simulink model "bh_lag_LQI_eom_quad_include_spin_props"  (R2021b)
settings: Solver=ode23t  StartTime=0.0  StopTime=200  FixedStep=0.001  RelTol=1e-5  EnableMultiTasking=on
values from neighbouring files (symbols this model uses):
  K = [1.17115605021e-19 -1.34457008772e-16 -7.12795123873e-18 0.0431836511993 -1.6541551896e-12 -1.73191982917e-16 0.126584124772 -3.94383892487e-18 1.65419671556e-12 0.126584124772 -1.82762947107e-16 -8.51651764895e-17 ... (60 elements, 4x15)]    [OLD_bh_CONT_DES_RESULTS_LQI_quadcopter.mat]    (also in bh_CONT_DES_RESULTS_LQI_quadcopter.mat = [2.6635655919e-18 -4.41749299763e-16 -1.11640474601e-16 0.04)
undefined symbols (not defined in the file or in its folder): P_elec, P_mot, P_one_prop, P_veh, sigbuilder_block
libraries: bh_6dof_LIBRARY x21, simulink_extras x12, slpidlib x4, simulink x1
(part 1 of 2)
settings Model: Creator=bhorton  LastModifiedBy=bhorton
settings SolverCC: AlgebraicLoopSolver=TrustRegion
settings DataIOCC: SaveOutput=off  SignalLogging=off  DSMLogging=off  VisualizeSimOutput=off  SaveTime=off  ReturnWorkspaceOutputs=off
settings OptimizationCC: LifeSpan=inf
settings DebuggingCC: AllowSymbolicDim=off  SFUnexpectedBacktrackingDiag=warning  SFNoUnconditionalDefaultTransitionDiag=warning  SFExecutionAtInitializationDiag=none  SFMachineParentedDataDiag=warning  ArithmeticOperatorsInVariantConditions=warning
settings ModelReferenceCC: PropagateSignalLabelsOutOfModel=off
settings SFSimCC: SimUseLocalCustomCode=off  CustomCodeUndefinedFunction=UseInterfaceOnly
settings RTWCC: RTWUseLocalCustomCode=off
settings CodeAppCC: StateflowObjectComments=on
settings GRTTargetCC: TargetLangStandard=C89/C90 (ANSI)
settings ConfigComp: CovMetricSettings=dw  CovSaveCumulativeToWorkspaceVar=on  CovSaveSingleToWorkspaceVar=on  CovExternalEMLEnable=off

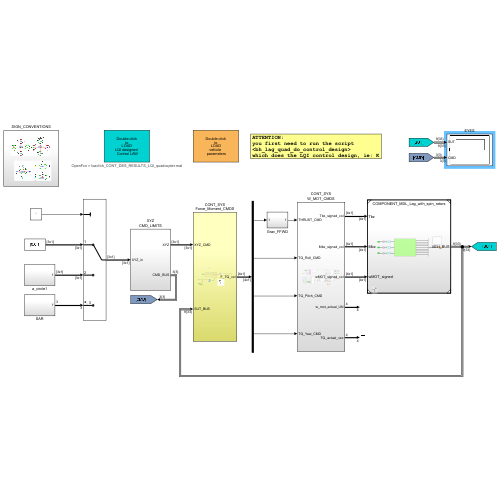
[thumbnail: Simulink's stored preview of the top-level diagram]
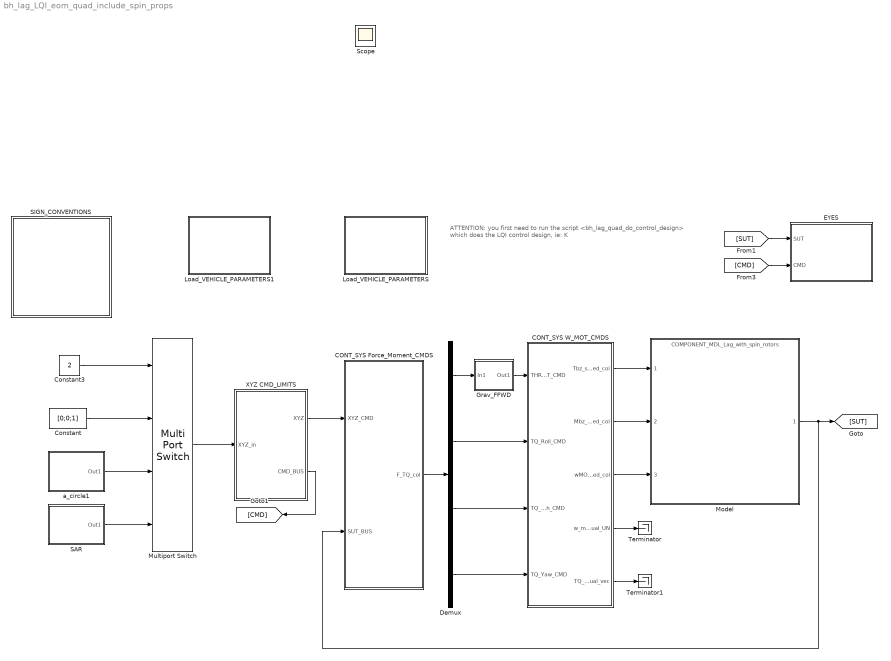
== system bh_lag_LQI_eom_quad_include_spin_props ==
  note: ATTENTION:
      | you first need to run the script
      | <bh_lag_quad_do_control_design>
      | which does the LQI control design, ie: K
  CONT_SYS Force_Moment_CMDS : Subsystem
  CONT_SYS W_MOT_CMDS : Subsystem
  Constant : Constant  Value=[0;0;1]  VectorParams1D=off
  Constant3 : Constant  Value=2
  Demux : Demux
  EYES : Subsystem
      mask Display: image('bh_PIC_SCOPE.jpg');
  Grav_FFWD : Subsystem
  Load_VEHICLE_PARAMETERS : Subsystem
      settings: OpenFcn=bh_create_local_params
      mask Display: disp('Double click\nto\nLOAD\nvehicle \n parameters')
  Load_VEHICLE_PARAMETERS1 : Subsystem
      settings: AttributesFormatString=OpenFcn = %<OpenFcn>  OpenFcn=load bh_CONT_DES_RESULTS_LQI_quadcopter.mat
      mask Display: disp('Double click\nto\nLOAD\nLQI designed \n Control LAW')
  Model : ModelReference  ModelNameDialog=COMPONENT_MDL_Lag_with_spin_rotors.slx  SimulationMode=Normal  ModelReferenceVersion=5.0
  Multiport Switch : MultiPortSwitch
  SAR : Subsystem
  SIGN_CONVENTIONS : Subsystem
  Terminator : Terminator
  Terminator1 : Terminator
  XYZ CMD_LIMITS : Subsystem
  a_circle1 : Subsystem
  Scope : Scope
  wires:
  [SUT] -> EYES/1(SUT)
  [CMD] -> EYES/2(CMD)
  XYZ CMD_LIMITS/1(XYZ) -> CONT_SYS Force_Moment_CMDS/1(XYZ_CMD)
  XYZ CMD_LIMITS/2(CMD_BUS) -> [CMD]
  CONT_SYS W_MOT_CMDS/4(w_mot_actual_UN) -> Terminator/1
  Model/1 -> CONT_SYS Force_Moment_CMDS/2(SUT_BUS), [SUT]
  CONT_SYS W_MOT_CMDS/3(wMOT_signed_col) -> Model/3
  CONT_SYS W_MOT_CMDS/5(TQ_actual_vec) -> Terminator1/1
  CONT_SYS W_MOT_CMDS/2(Mbz_signed_col) -> Model/2
  CONT_SYS W_MOT_CMDS/1(Tbz_signed_col) -> Model/1
  CONT_SYS Force_Moment_CMDS/1(F_TQ_col) -> Demux/1
  Demux/2 -> CONT_SYS W_MOT_CMDS/2(TQ_Roll_CMD)
  Demux/3 -> CONT_SYS W_MOT_CMDS/3(TQ_Pitch_CMD)
  Demux/4 -> CONT_SYS W_MOT_CMDS/4(TQ_Yaw_CMD)
  Constant/1 -> Multiport Switch/2
  Constant3/1 -> Multiport Switch/1
  SAR/1(Out1) -> Multiport Switch/4
  a_circle1/1(Out1) -> Multiport Switch/3
  Multiport Switch/1 -> XYZ CMD_LIMITS/1(XYZ_in)
  Demux/1 -> Grav_FFWD/1(In1)
  Grav_FFWD/1(Out1) -> CONT_SYS W_MOT_CMDS/1(THRUST_CMD)

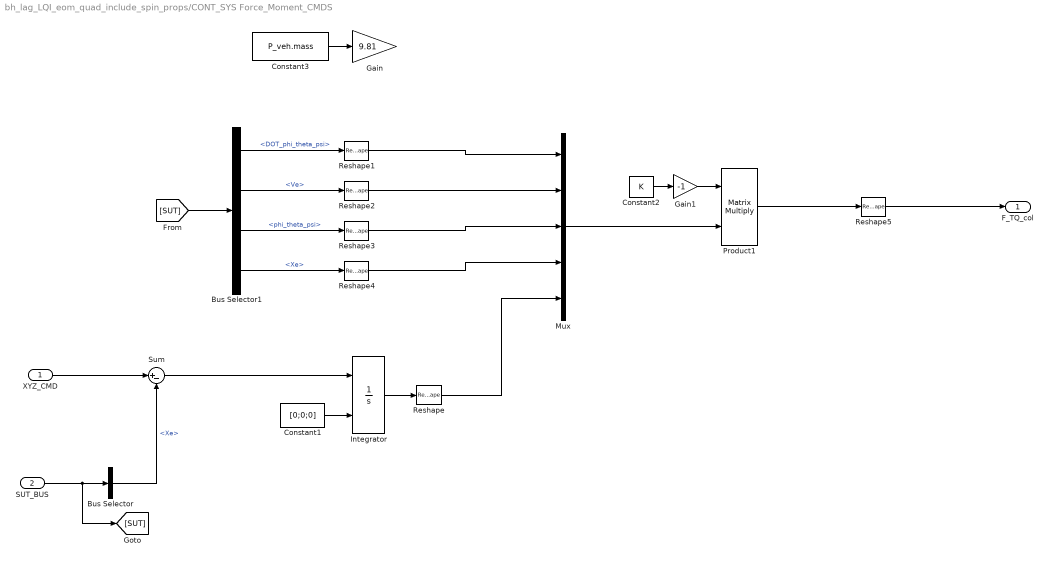
== system bh_lag_LQI_eom_quad_include_spin_props/CONT_SYS Force_Moment_CMDS ==
  XYZ_CMD : Inport
  SUT_BUS : Inport  Port=2
  Bus Selector : BusSelector  OutputSignals=Xe
  Bus Selector1 : BusSelector  OutputSignals=DOT_phi_theta_psi,Ve,phi_theta_psi,Xe
  Constant1 : Constant  Value=[0;0;0]  VectorParams1D=off
  Constant2 : Constant  Value=K  VectorParams1D=off
  Constant3 : Constant  Value=P_veh.mass
  Gain : Gain  Gain=9.81
  Gain1 : Gain  Gain=-1
  Integrator : Integrator  InitialConditionSource=external
  Mux : Mux  Inputs=5
  Product1 : Product  Multiplication=Matrix(*)
  Reshape{,1..5} (6 alike) : Reshape  OutputDimensionality=Column vector (2-D)
  Sum : Sum  Inputs=|+-
  F_TQ_col : Outport  VectorParamsAs1DForOutWhenUnconnected=off
  wires:
  SUT_BUS/1 -> [SUT], Bus Selector/1
  Constant3/1 -> Gain/1
  Constant1/1 -> Integrator/2
  Integrator/1 -> Reshape/1
  Reshape/1 -> Mux/5
  XYZ_CMD/1 -> Sum/1
  Sum/1 -> Integrator/1
  Bus Selector/1 -> Sum/2  "<Xe>"
  [SUT] -> Bus Selector1/1
  Bus Selector1/1 -> Reshape1/1  "<DOT_phi_theta_psi>"
  Bus Selector1/2 -> Reshape2/1  "<Ve>"
  Bus Selector1/3 -> Reshape3/1  "<phi_theta_psi>"
  Bus Selector1/4 -> Reshape4/1  "<Xe>"
  Reshape1/1 -> Mux/1
  Reshape2/1 -> Mux/2
  Reshape3/1 -> Mux/3
  Reshape4/1 -> Mux/4
  Constant2/1 -> Gain1/1
  Gain1/1 -> Product1/1
  Mux/1 -> Product1/2
  Product1/1 -> Reshape5/1
  Reshape5/1 -> F_TQ_col/1

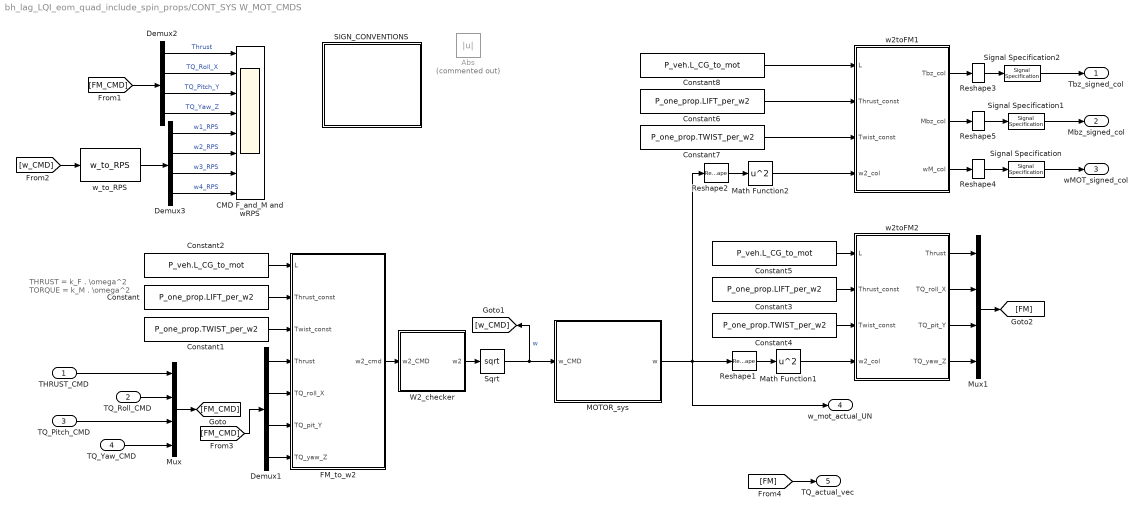
== system bh_lag_LQI_eom_quad_include_spin_props/CONT_SYS W_MOT_CMDS ==
  note: THRUST = k_F . \omega^2
      |
      | TORQUE = k_M . \omega^2
  THRUST_CMD : Inport
  TQ_Roll_CMD : Inport  Port=2
  TQ_Pitch_CMD : Inport  Port=3
  TQ_Yaw_CMD : Inport  Port=4
  Abs : Abs  Commented=on
  CMD F_and_M and wRPS : Scope  NumInputPorts=8
  Constant : Constant  Value=P_one_prop.LIFT_per_w2
  Constant1 : Constant  Value=P_one_prop.TWIST_per_w2
  Constant2 : Constant  Value=P_veh.L_CG_to_mot
  Constant3 : Constant  Value=P_one_prop.LIFT_per_w2
  Constant4 : Constant  Value=P_one_prop.TWIST_per_w2
  Constant5 : Constant  Value=P_veh.L_CG_to_mot
  Constant6 : Constant  Value=P_one_prop.LIFT_per_w2
  Constant7 : Constant  Value=P_one_prop.TWIST_per_w2
  Constant8 : Constant  Value=P_veh.L_CG_to_mot
  Demux1 : Demux
  Demux2 : Demux
  Demux3 : Demux
  FM_to_w2 : MATLAB Function  TreatAsAtomicUnit=on
  MOTOR_sys : Subsystem
      mask Display: image('bh_PIC_MOTOR.jpg');
  Math Function1 : Math  Operator=square  SignedPower=on  SaturateOnIntegerOverflow=on
  Math Function2 : Math  Operator=square  SignedPower=on  SaturateOnIntegerOverflow=on
  Mux : Mux
  Mux1 : Mux
  Reshape{1..5} (5 alike) : Reshape  OutputDimensionality=Column vector (2-D)
  SIGN_CONVENTIONS : Subsystem
  Signal Specification : SignalSpecification  Dimensions=[4,1]
  Signal Specification1 : SignalSpecification  Dimensions=[4,1]
  Signal Specification2 : SignalSpecification  Dimensions=[4,1]
  Sqrt : Sqrt  SaturateOnIntegerOverflow=on
  W2_checker : Subsystem
  w2toFM1 : MATLAB Function  TreatAsAtomicUnit=on
  w2toFM2 : MATLAB Function  TreatAsAtomicUnit=on
  w_to_RPS : bh_6dof_LIBRARY/MODELS/w_to_RPS  SystemSampleTime=-1  VariantActivationTime=update diagram  Latency=0  AutoFrameSizeCalculation=off
  Tbz_signed_col : Outport  VectorParamsAs1DForOutWhenUnconnected=off
  Mbz_signed_col : Outport  Port=2  VectorParamsAs1DForOutWhenUnconnected=off
  wMOT_signed_col : Outport  Port=3  VectorParamsAs1DForOutWhenUnconnected=off
  w_mot_actual_UN : Outport  Port=4  VectorParamsAs1DForOutWhenUnconnected=off
  TQ_actual_vec : Outport  Port=5  VectorParamsAs1DForOutWhenUnconnected=off
  wires:
  Constant1/1 -> FM_to_w2/3(Twist_const)
  Constant/1 -> FM_to_w2/2(Thrust_const)
  Constant2/1 -> FM_to_w2/1(L)
  Sqrt/1 -> MOTOR_sys/1(w_CMD), [w_CMD]  "w"
  W2_checker/1(w2) -> Sqrt/1
  Demux1/1 -> FM_to_w2/4(Thrust)
  Demux1/2 -> FM_to_w2/5(TQ_roll_X)
  Demux1/3 -> FM_to_w2/6(TQ_pit_Y)
  Demux1/4 -> FM_to_w2/7(TQ_yaw_Z)
  THRUST_CMD/1 -> Mux/1
  TQ_Roll_CMD/1 -> Mux/2
  TQ_Pitch_CMD/1 -> Mux/3
  TQ_Yaw_CMD/1 -> Mux/4
  Mux/1 -> [FM_CMD]
  [FM_CMD] -> Demux1/1
  Demux2/1 -> CMD F_and_M and wRPS/1  "Thrust"
  Demux2/2 -> CMD F_and_M and wRPS/2  "TQ_Roll_X"
  Demux2/3 -> CMD F_and_M and wRPS/3  "TQ_Pitch_Y"
  Demux2/4 -> CMD F_and_M and wRPS/4  "TQ_Yaw_Z"
  Demux3/2 -> CMD F_and_M and wRPS/6  "w2_RPS"
  Demux3/1 -> CMD F_and_M and wRPS/5  "w1_RPS"
  Demux3/4 -> CMD F_and_M and wRPS/8  "w4_RPS"
  Demux3/3 -> CMD F_and_M and wRPS/7  "w3_RPS"
  [FM_CMD] -> Demux2/1
  w_to_RPS/1 -> Demux3/1
  [w_CMD] -> w_to_RPS/1
  Constant3/1 -> w2toFM2/2(Thrust_const)
  Constant4/1 -> w2toFM2/3(Twist_const)
  Constant5/1 -> w2toFM2/1(L)
  Mux1/1 -> [FM]
  Reshape1/1 -> Math Function1/1
  Math Function1/1 -> w2toFM2/4(w2_col)
  [FM] -> TQ_actual_vec/1
  w2toFM2/1(Thrust) -> Mux1/1
  w2toFM2/2(TQ_roll_X) -> Mux1/2
  w2toFM2/3(TQ_pit_Y) -> Mux1/3
  w2toFM2/4(TQ_yaw_Z) -> Mux1/4
  Reshape2/1 -> Math Function2/1
  Math Function2/1 -> w2toFM1/4(w2_col)
  Constant7/1 -> w2toFM1/3(Twist_const)
  Constant6/1 -> w2toFM1/2(Thrust_const)
  Constant8/1 -> w2toFM1/1(L)
  w2toFM1/2(Mbz_col) -> Reshape5/1
  w2toFM1/1(Tbz_col) -> Reshape3/1
  w2toFM1/3(wM_col) -> Reshape4/1
  Reshape3/1 -> Signal Specification2/1
  Reshape5/1 -> Signal Specification1/1
  Reshape4/1 -> Signal Specification/1
  Signal Specification2/1 -> Tbz_signed_col/1
  Signal Specification1/1 -> Mbz_signed_col/1
  Signal Specification/1 -> wMOT_signed_col/1
  FM_to_w2/1(w2_cmd) -> W2_checker/1(w2_CMD)
  MOTOR_sys/1(w) -> Reshape1/1, w_mot_actual_UN/1, Reshape2/1

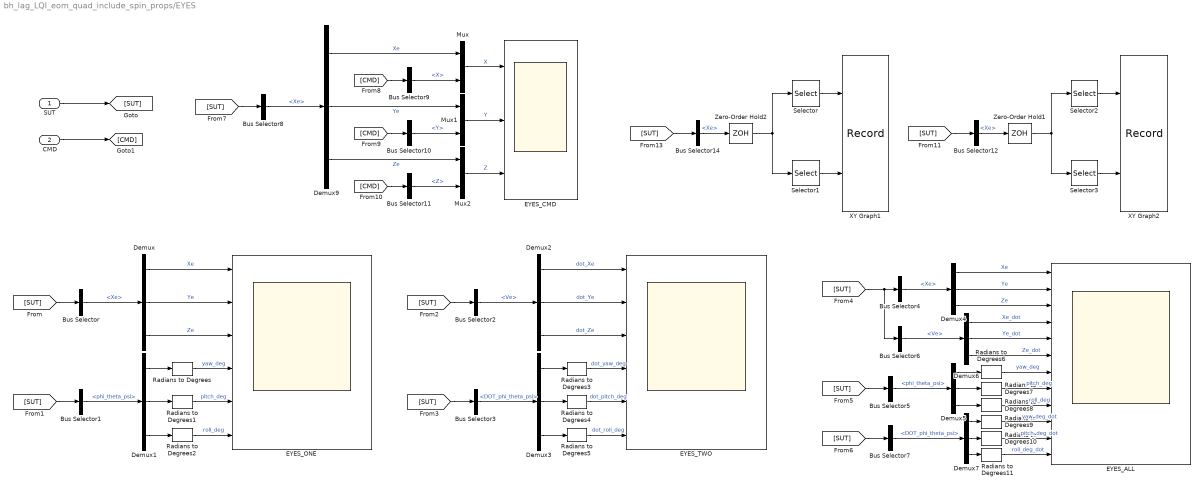
== system bh_lag_LQI_eom_quad_include_spin_props/EYES ==
  SUT : Inport
  CMD : Inport  Port=2
  Bus Selector{,4,8,12,14} (5 alike) : BusSelector  OutputSignals=Xe
  Bus Selector1 : BusSelector  OutputSignals=phi_theta_psi
  Bus Selector10 : BusSelector  OutputSignals=Y
  Bus Selector11 : BusSelector  OutputSignals=Z
  Bus Selector2 : BusSelector  OutputSignals=Ve
  Bus Selector3 : BusSelector  OutputSignals=DOT_phi_theta_psi
  Bus Selector5 : BusSelector  OutputSignals=phi_theta_psi
  Bus Selector6 : BusSelector  OutputSignals=Ve
  Bus Selector7 : BusSelector  OutputSignals=DOT_phi_theta_psi
  Bus Selector9 : BusSelector  OutputSignals=X
  Demux{,1..7,9} (9 alike) : Demux  Outputs=3
  EYES_ALL : Scope  NumInputPorts=12
  EYES_CMD : Scope  NumInputPorts=3
  EYES_ONE : Scope  NumInputPorts=6
  EYES_TWO : Scope  NumInputPorts=6
  Mux : Mux  Inputs=2
  Mux1 : Mux  Inputs=2
  Mux2 : Mux  Inputs=2
  Radians to Degrees{,1..11} (12 alike) : simulink_extras/Transformations/Radians to Degrees
  Selector : Selector  InputPortWidth=3  IndexOptions=Index vector (dialog)  Indices=1  OutputSizes=1
  Selector1 : Selector  InputPortWidth=3  IndexOptions=Index vector (dialog)  Indices=2  OutputSizes=1
  Selector2 : Selector  InputPortWidth=3  IndexOptions=Index vector (dialog)  Indices=1  OutputSizes=1
  Selector3 : Selector  InputPortWidth=3  IndexOptions=Index vector (dialog)  Indices=2  OutputSizes=1
  XY Graph1 : Record  FileSettingsInternal="{\"entries\":[{\"content\":{\"excelSettings\":{\"content\":{},\"type\":\"Streamout.ExcelSettings\"}},\"type\":\"Streamout.FileSettingStorage\",\"uuid\":\"a83ad9bf-e0f6-43ab-9986-ce40615f0ff9\"}],\"packageUris\":[\"http://schema.mathworks.com/mf0/streamout_blocks/R2020a\"],\"version\":\"1.0\"}"  Layout=[1 1]  SignalsInternal="{\"entries\":[{\"content\":{\"signals\":[{\"content\":{\"blockPath\":[\"bh_lag_LQI_eom_quad_include_spin_props/EYES/XY Graph1\"],\"channel\":[],\"dimensions\":[1,1],\"domain\":\"bh_lag_LQI_eom_quad_include_spin_props/EYES/XY Graph1\",\"lineColor\":\"#a2142f\",\"plots\":[1],\"port\":1,\"sid\":[\"\"],\"signalID\":12934,\"signalName\":\"Selector\"},\"type\":\"RecordBlkView.Signal\",\"uuid\":\"290329af-9585-46bd-91fa-6e542c395c0f\"},{\"content\":{\"blockPath\":[\"bh_lag_LQI_eom_quad_include_spin_props/EYES/XY Graph1\"],\"channel\":[],\"dimensions\":[1,1],\"domain\":\"bh_lag_LQI_eom_quad_include_spin_props/EYES/XY Graph1\",\"lineColor\":\"#139fff\",\"plots\":[1],\"port\":2,\"sid\":[\"\"],\"signalID\":12938,\"signalName\":\"Selector1\"},\"type\":\"RecordBlkView.Signal\",\"uuid\":\"d59bf6d2-ff61-4869-8b7a-6463b592cd81\"}]},\"type\":\"RecordBlkView.InputSignals\",\"uuid\":\"1ae0fd58-1ec5-45c4-96f2-b1e491a41671\"}],\"packageUris\":[\"http://schema.mathworks.com/mf0/streamout_blocks/R2020a\"],\"version\":\"1.0\"}"  VisualizationBindings="{\"xyplotplugin\":{\"info\":[{\"series\":[{\"bindingParametersList\":[{\"parameter\":\"X-Axis\",\"signalID\":12934,\"signalName\":\"Selector\"},{\"parameter\":\"Y-Axis\",\"signalID\":12938,\"signalName\":\"Selector1\"}],\"seriesID\":26532}],\"subplotID\":1}]}}"  CompatibilityTag=XY  st=-1
  XY Graph2 : Record  FileSettingsInternal="{\"entries\":[{\"content\":{\"excelSettings\":{\"content\":{},\"type\":\"Streamout.ExcelSettings\"}},\"type\":\"Streamout.FileSettingStorage\",\"uuid\":\"bc2f2a3d-5443-46df-af74-32db6837a512\"}],\"packageUris\":[\"http://schema.mathworks.com/mf0/streamout_blocks/R2020a\"],\"version\":\"1.0\"}"  Layout=[1 1]  SignalsInternal="{\"entries\":[{\"content\":{\"signals\":[{\"content\":{\"blockPath\":[\"bh_lag_LQI_eom_quad_include_spin_props/EYES/XY Graph2\"],\"channel\":[],\"dimensions\":[1,1],\"domain\":\"bh_lag_LQI_eom_quad_include_spin_props/EYES/XY Graph2\",\"lineColor\":\"#a2142f\",\"plots\":[1],\"port\":1,\"sid\":[\"\"],\"signalID\":12942,\"signalName\":\"Selector2\"},\"type\":\"RecordBlkView.Signal\",\"uuid\":\"1ef547bc-a7a6-4f16-8c37-dae7699654e6\"},{\"content\":{\"blockPath\":[\"bh_lag_LQI_eom_quad_include_spin_props/EYES/XY Graph2\"],\"channel\":[],\"dimensions\":[1,1],\"domain\":\"bh_lag_LQI_eom_quad_include_spin_props/EYES/XY Graph2\",\"lineColor\":\"#139fff\",\"plots\":[1],\"port\":2,\"sid\":[\"\"],\"signalID\":12946,\"signalName\":\"Selector3\"},\"type\":\"RecordBlkView.Signal\",\"uuid\":\"3af2e148-9d5b-4cdb-a3d4-2d95b89efa31\"}]},\"type\":\"RecordBlkView.InputSignals\",\"uuid\":\"e4d7a602-e7ea-4692-b35f-6ef19b620167\"}],\"packageUris\":[\"http://schema.mathworks.com/mf0/streamout_blocks/R2020a\"],\"version\":\"1.0\"}"  VisualizationBindings="{\"xyplotplugin\":{\"info\":[{\"series\":[{\"bindingParametersList\":[{\"parameter\":\"X-Axis\",\"signalID\":12942,\"signalName\":\"Selector2\"},{\"parameter\":\"Y-Axis\",\"signalID\":12946,\"signalName\":\"Selector3\"}],\"seriesID\":9493}],\"subplotID\":1}]}}"  CompatibilityTag=XY  st=-1
  Zero-Order Hold1 : ZeroOrderHold  SampleTime=0.1
  Zero-Order Hold2 : ZeroOrderHold  SampleTime=0.1
  wires:
  SUT/1 -> [SUT]
  [SUT] -> Bus Selector/1
  Demux/2 -> EYES_ONE/2  "Ye"
  Demux/3 -> EYES_ONE/3  "Ze"
  Demux/1 -> EYES_ONE/1  "Xe"
  Bus Selector/1 -> Demux/1  "<Xe>"
  Bus Selector1/1 -> Demux1/1  "<phi_theta_psi>"
  [SUT] -> Bus Selector1/1
  Demux1/1 -> Radians to Degrees/1
  Radians to Degrees/1 -> EYES_ONE/4  "yaw_deg"
  Radians to Degrees1/1 -> EYES_ONE/5  "pitch_deg"
  Radians to Degrees2/1 -> EYES_ONE/6  "roll_deg"
  Demux1/3 -> Radians to Degrees2/1
  Demux1/2 -> Radians to Degrees1/1
  [SUT] -> Bus Selector2/1
  Demux2/2 -> EYES_TWO/2  "dot_Ye"
  Demux2/3 -> EYES_TWO/3  "dot_Ze"
  Demux2/1 -> EYES_TWO/1  "dot_Xe"
  Bus Selector2/1 -> Demux2/1  "<Ve>"
  Bus Selector3/1 -> Demux3/1  "<DOT_phi_theta_psi>"
  [SUT] -> Bus Selector3/1
  Demux3/1 -> Radians to Degrees3/1
  Radians to Degrees3/1 -> EYES_TWO/4  "dot_yaw_deg"
  Radians to Degrees4/1 -> EYES_TWO/5  "dot_pitch_deg"
  Radians to Degrees5/1 -> EYES_TWO/6  "dot_roll_deg"
  Demux3/3 -> Radians to Degrees5/1
  Demux3/2 -> Radians to Degrees4/1
  [SUT] -> Bus Selector6/1, Bus Selector4/1
  Demux4/2 -> EYES_ALL/2  "Ye"
  Demux4/3 -> EYES_ALL/3  "Ze"
  Demux4/1 -> EYES_ALL/1  "Xe"
  Bus Selector4/1 -> Demux4/1  "<Xe>"
  Bus Selector5/1 -> Demux5/1  "<phi_theta_psi>"
  [SUT] -> Bus Selector5/1
  Demux5/1 -> Radians to Degrees6/1
  Demux6/1 -> EYES_ALL/4  "Xe_dot"
  Demux6/2 -> EYES_ALL/5  "Ye_dot"
  Demux6/3 -> EYES_ALL/6  "Ze_dot"
  Demux5/3 -> Radians to Degrees8/1
  Demux5/2 -> Radians to Degrees7/1
  Bus Selector6/1 -> Demux6/1  "<Ve>"
  Radians to Degrees6/1 -> EYES_ALL/7  "yaw_deg"
  Radians to Degrees7/1 -> EYES_ALL/8  "pitch_deg"
  Radians to Degrees8/1 -> EYES_ALL/9  "roll_deg"
  Bus Selector7/1 -> Demux7/1  "<DOT_phi_theta_psi>"
  [SUT] -> Bus Selector7/1
  Demux7/1 -> Radians to Degrees9/1
  Demux7/2 -> Radians to Degrees10/1
  Demux7/3 -> Radians to Degrees11/1
  Radians to Degrees9/1 -> EYES_ALL/10  "yaw_deg_dot"
  Radians to Degrees10/1 -> EYES_ALL/11  "pitch_deg_dot"
  Radians to Degrees11/1 -> EYES_ALL/12  "roll_deg_dot"
  CMD/1 -> [CMD]
  [SUT] -> Bus Selector8/1
  Demux9/2 -> Mux1/1  "Ye"
  Demux9/1 -> Mux/1  "Xe"
  Bus Selector8/1 -> Demux9/1  "<Xe>"
  Mux/1 -> EYES_CMD/1  "X"
  Mux1/1 -> EYES_CMD/2  "Y"
  Mux2/1 -> EYES_CMD/3  "Z"
  Demux9/3 -> Mux2/1  "Ze"
  [CMD] -> Bus Selector9/1
  Bus Selector9/1 -> Mux/2  "<X>"
  [CMD] -> Bus Selector10/1
  Bus Selector10/1 -> Mux1/2  "<Y>"
  [CMD] -> Bus Selector11/1
  Bus Selector11/1 -> Mux2/2  "<Z>"
  [SUT] -> Bus Selector14/1
  Bus Selector14/1 -> Zero-Order Hold2/1  "<Xe>"
  Zero-Order Hold2/1 -> Selector1/1, Selector/1
  Selector1/1 -> XY Graph1/2
  Selector/1 -> XY Graph1/1
  [SUT] -> Bus Selector12/1
  Zero-Order Hold1/1 -> Selector3/1, Selector2/1
  Selector3/1 -> XY Graph2/2
  Selector2/1 -> XY Graph2/1
  Bus Selector12/1 -> Zero-Order Hold1/1  "<Xe>"

== system bh_lag_LQI_eom_quad_include_spin_props/Grav_FFWD ==
  In1 : Inport
  Constant3 : Constant  Value=P_veh.mass
  Gain : Gain  Gain=9.81
  Sum : Sum  Inputs=++|
  Out1 : Outport  VectorParamsAs1DForOutWhenUnconnected=off
  wires:
  Gain/1 -> Sum/1
  Constant3/1 -> Gain/1
  Sum/1 -> Out1/1
  In1/1 -> Sum/2

== system bh_lag_LQI_eom_quad_include_spin_props/Load_VEHICLE_PARAMETERS ==

== system bh_lag_LQI_eom_quad_include_spin_props/Load_VEHICLE_PARAMETERS1 ==

== system bh_lag_LQI_eom_quad_include_spin_props/SAR ==
  Mux : Mux  Inputs=3
  Selector : Selector  InputPortWidth=3  IndexOptions=Index vector (dialog)  Indices=[2 3 1]  OutputSizes=1
  XYZ_CMDS : Subsystem  Tag=STV Subsys  LoadFcn=sigbuilder_block('load');  StartFcn=sigbuilder_block('start');  StopFcn=sigbuilder_block('stop');  ClipboardFcn=sigbuilder_block('clipboard');  mask(Sigbuilder block){tuvar=[0:10]}
      mask help: Simulink:masks:SigbuilderBlock_MD
      mask init:
      | if ~strcmp(get_param(bdroot(gcbh),'SimulationStatus'),'stopped') tuvar = sigbuilder_block('maskInit'); end
      settings: CopyFcn=sigbuilder_block('copy');  DeleteFcn=sigbuilder_block('delete');  ModelCloseFcn=sigbuilder_block('modelClose');  PreSaveFcn=sigbuilder_block('preSave');  PauseFcn=sigbuilder_block('pause');  ContinueFcn=sigbuilder_block('continue');  NameChangeFcn=sigbuilder_block('namechange');  OpenFcn=sigbuilder_block('open',[189 32.25 551.25 400.5 ]);  CloseFcn=sigbuilder_block('close');
      mask Display: plot(0, 0, 100, 100,[2, 2, 32, 32, 2], [68, 8, 8, 68, 68],[32, 2], [38, 38], [32, 19, 2],[53, 60, 44], [32, 17, 17, 2],[16, 16, 31, 31]);txt = getActiveGroup(gcbh);text(2, 100, txt,'verticalAlignment', 'top');
  Out1 : Outport  VectorParamsAs1DForOutWhenUnconnected=off
  wires:
  XYZ_CMDS/3(Y) -> Mux/3
  XYZ_CMDS/1(Z) -> Mux/1
  XYZ_CMDS/2(X) -> Mux/2
  Mux/1 -> Selector/1
  Selector/1 -> Out1/1

== system bh_lag_LQI_eom_quad_include_spin_props/SIGN_CONVENTIONS ==

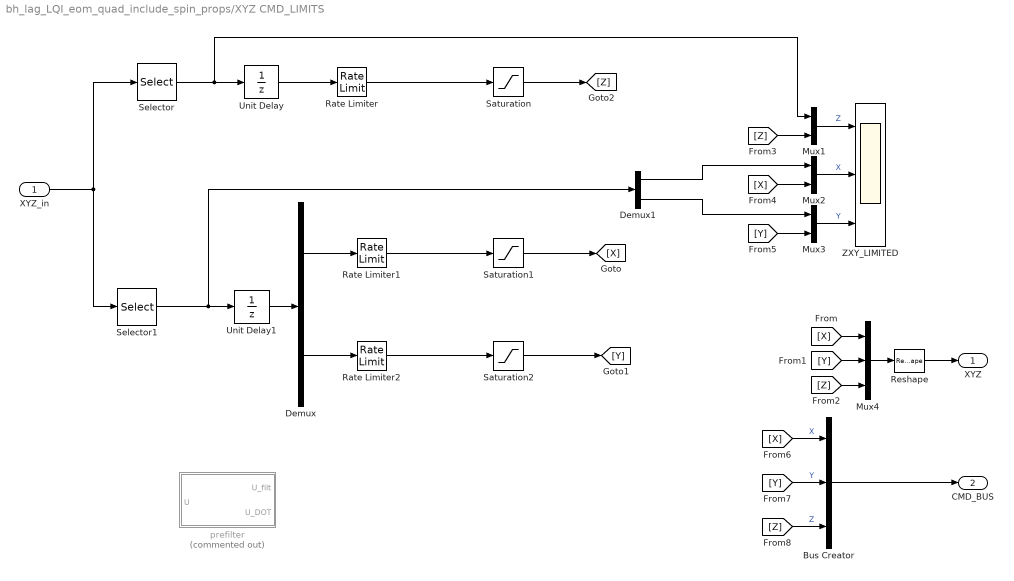
== system bh_lag_LQI_eom_quad_include_spin_props/XYZ CMD_LIMITS ==
  XYZ_in : Inport
  Bus Creator : BusCreator  Inputs=3
  Demux : Demux  Outputs=2
  Demux1 : Demux  Outputs=2
  Mux1 : Mux  Inputs=2
  Mux2 : Mux  Inputs=2
  Mux3 : Mux  Inputs=2
  Mux4 : Mux  Inputs=3
  Rate Limiter : RateLimiter  RisingSlewLimit=2  FallingSlewLimit=-2
      settings: AttributesFormatString=|
      | Rising_rate = %<RisingSlewLimit>
      | Falling_rate = %<FallingSlewLimit>
  Rate Limiter1 : RateLimiter  RisingSlewLimit=3  FallingSlewLimit=-3
      settings: AttributesFormatString=|
      | Rising_rate = %<RisingSlewLimit>
      | Falling_rate = %<FallingSlewLimit>
  Rate Limiter2 : RateLimiter  RisingSlewLimit=3  FallingSlewLimit=-3
      settings: AttributesFormatString=|
      | Rising_rate = %<RisingSlewLimit>
      | Falling_rate = %<FallingSlewLimit>
  Reshape : Reshape  OutputDimensionality=Column vector (2-D)
  Saturation : Saturate  UpperLimit=500  LowerLimit=0
      settings: AttributesFormatString=|
      | MAX =    %<UpperLimit>
      | MIN = %<LowerLimit>
  Saturation1 : Saturate  UpperLimit=500  LowerLimit=-500
      settings: AttributesFormatString=|
      | MAX =    %<UpperLimit>
      | MIN = %<LowerLimit>
  Saturation2 : Saturate  UpperLimit=500  LowerLimit=-500
      settings: AttributesFormatString=|
      | MAX =    %<UpperLimit>
      | MIN = %<LowerLimit>
  Selector : Selector  InputPortWidth=3  IndexOptions=Index vector (dialog)  Indices=3  OutputSizes=1
  Selector1 : Selector  InputPortWidth=3  IndexOptions=Index vector (dialog)  Indices=[1 2]  OutputSizes=1
  Unit Delay : UnitDelay  SampleTime=0.01  HasFrameUpgradeWarning=on
  Unit Delay1 : UnitDelay  SampleTime=0.01  HasFrameUpgradeWarning=on
  ZXY_LIMITED : Scope  NumInputPorts=3
  prefilter : Subsystem  Commented=on  mask(Derivative Estimation){wn=2*pi*0.5, p=1}
      mask prompts: wn "Natural frequency, wn (rad/sec)"; p "Damping ratio, p"
      mask help:
      | A simple derivative estimator using a 2nd order representation between input and output.
      |
      | The integrators use a discrete FORWARd Euler rule, and a sample time needs to be specified.
      mask init:
      | str1 = sprintf('wn = %.2f', wn);
      | str2 = sprintf('p  = %.2f', p);
      | %str3 = sprintf('dt = %.2f', dt);
      | %str = char(str1,str2,str3);
      | %str3 = sprintf('dt = %.2f', dt);
      | str = char(str1,str2);
      mask Display: disp(str)
  XYZ : Outport  VectorParamsAs1DForOutWhenUnconnected=off
  CMD_BUS : Outport  Port=2  VectorParamsAs1DForOutWhenUnconnected=off
  wires:
  Selector1/1 -> Demux1/1, Unit Delay1/1
  Demux/1 -> Rate Limiter1/1
  Demux/2 -> Rate Limiter2/1
  Saturation1/1 -> [X]
  Saturation2/1 -> [Y]
  Mux4/1 -> Reshape/1
  Selector/1 -> Mux1/1, Unit Delay/1
  Rate Limiter/1 -> Saturation/1
  Unit Delay/1 -> Rate Limiter/1
  Unit Delay1/1 -> Demux/1
  Rate Limiter1/1 -> Saturation1/1
  Rate Limiter2/1 -> Saturation2/1
  [X] -> Mux4/1
  [Y] -> Mux4/2
  [Z] -> Mux4/3
  Saturation/1 -> [Z]
  [Z] -> Mux1/2
  [Y] -> Mux3/2
  Demux1/1 -> Mux2/1
  Demux1/2 -> Mux3/1
  [X] -> Mux2/2
  Mux1/1 -> ZXY_LIMITED/1  "Z"
  Mux2/1 -> ZXY_LIMITED/2  "X"
  Mux3/1 -> ZXY_LIMITED/3  "Y"
  Bus Creator/1 -> CMD_BUS/1
  [Y] -> Bus Creator/2  "Y"
  [X] -> Bus Creator/1  "X"
  [Z] -> Bus Creator/3  "Z"
  Reshape/1 -> XYZ/1
  XYZ_in/1 -> Selector1/1, Selector/1

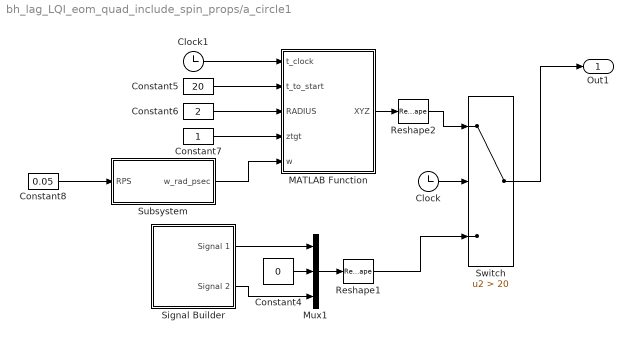
== system bh_lag_LQI_eom_quad_include_spin_props/a_circle1 ==
  Clock : Clock
  Clock1 : Clock
  Constant4 : Constant  Value=0  VectorParams1D=off
  Constant5 : Constant  Value=20  VectorParams1D=off
  Constant6 : Constant  Value=2  VectorParams1D=off
  Constant7 : Constant  VectorParams1D=off
  Constant8 : Constant  Value=0.05  VectorParams1D=off
  MATLAB Function : MATLAB Function  TreatAsAtomicUnit=on
  Mux1 : Mux  Inputs=3
  Reshape1 : Reshape  OutputDimensionality=Column vector (2-D)
  Reshape2 : Reshape  OutputDimensionality=Column vector (2-D)
  Signal Builder : Subsystem  Tag=STV Subsys  LoadFcn=sigbuilder_block('load');  StartFcn=sigbuilder_block('start');  StopFcn=sigbuilder_block('stop');  ClipboardFcn=sigbuilder_block('clipboard');  mask(Sigbuilder block){tuvar=[0:10]}
      mask help: Simulink:masks:SigbuilderBlock_MD
      mask init:
      | if ~strcmp(get_param(bdroot(gcbh),'SimulationStatus'),'stopped') tuvar = sigbuilder_block('maskInit'); end
      settings: CopyFcn=sigbuilder_block('copy');  DeleteFcn=sigbuilder_block('delete');  ModelCloseFcn=sigbuilder_block('modelClose');  PreSaveFcn=sigbuilder_block('preSave');  PauseFcn=sigbuilder_block('pause');  ContinueFcn=sigbuilder_block('continue');  NameChangeFcn=sigbuilder_block('namechange');  OpenFcn=sigbuilder_block('open',[437.6 199.2 550.4 400 ]);  CloseFcn=sigbuilder_block('close');
      mask Display: plot(0, 0, 100, 100,[2, 2, 32, 32, 2], [68, 8, 8, 68, 68],[32, 2], [38, 38], [32, 19, 2],[53, 60, 44], [32, 17, 17, 2],[16, 16, 31, 31]);txt = getActiveGroup(gcbh);text(2, 100, txt,'verticalAlignment', 'top');
  Subsystem : Subsystem
  Switch : Switch  Criteria=u2 > Threshold  Threshold=20
  Out1 : Outport  VectorParamsAs1DForOutWhenUnconnected=off
  wires:
  Switch/1 -> Out1/1
  MATLAB Function/1(XYZ) -> Reshape2/1
  Constant6/1 -> MATLAB Function/3(RADIUS)
  Constant7/1 -> MATLAB Function/4(ztgt)
  Subsystem/1(w_rad_psec) -> MATLAB Function/5(w)
  Constant5/1 -> MATLAB Function/2(t_to_start)
  Reshape1/1 -> Switch/3
  Constant4/1 -> Mux1/2
  Signal Builder/1(Signal 1) -> Mux1/1
  Signal Builder/2(Signal 2) -> Mux1/3
  Mux1/1 -> Reshape1/1
  Clock/1 -> Switch/2
  Clock1/1 -> MATLAB Function/1(t_clock)
  Constant8/1 -> Subsystem/1(RPS)
  Reshape2/1 -> Switch/1

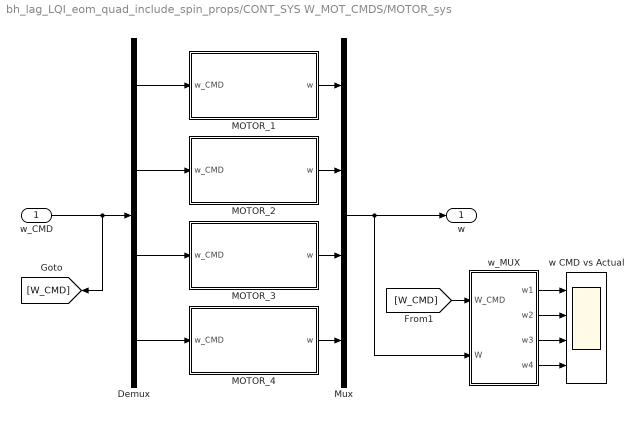
== system bh_lag_LQI_eom_quad_include_spin_props/CONT_SYS W_MOT_CMDS/MOTOR_sys ==
  w_CMD : Inport
  Demux : Demux
  MOTOR_1 : Subsystem
      mask Display: image('bh_PIC_MOTOR.jpg');
  MOTOR_2 : Subsystem
      mask Display: image('bh_PIC_MOTOR.jpg');
  MOTOR_3 : Subsystem
      mask Display: image('bh_PIC_MOTOR.jpg');
  MOTOR_4 : Subsystem
      mask Display: image('bh_PIC_MOTOR.jpg');
  Mux : Mux
  w CMD vs Actual : Scope  NumInputPorts=4
  w_MUX : Subsystem
  w : Outport  VectorParamsAs1DForOutWhenUnconnected=off
  wires:
  MOTOR_4/1(w) -> Mux/4
  MOTOR_3/1(w) -> Mux/3
  MOTOR_2/1(w) -> Mux/2
  MOTOR_1/1(w) -> Mux/1
  Demux/1 -> MOTOR_1/1(w_CMD)
  Demux/2 -> MOTOR_2/1(w_CMD)
  Demux/3 -> MOTOR_3/1(w_CMD)
  Demux/4 -> MOTOR_4/1(w_CMD)
  w_CMD/1 -> [W_CMD], Demux/1
  w_MUX/4(w4) -> w CMD vs Actual/4
  w_MUX/2(w2) -> w CMD vs Actual/2
  w_MUX/3(w3) -> w CMD vs Actual/3
  w_MUX/1(w1) -> w CMD vs Actual/1
  [W_CMD] -> w_MUX/1(W_CMD)
  Mux/1 -> w_MUX/2(W), w/1

== system bh_lag_LQI_eom_quad_include_spin_props/CONT_SYS W_MOT_CMDS/SIGN_CONVENTIONS ==

== system bh_lag_LQI_eom_quad_include_spin_props/CONT_SYS W_MOT_CMDS/W2_checker ==
  w2_CMD : Inport
  Assertion{,1..3} (4 alike) : Assertion
  Compare To Constant : simulink/Logic and Bit Operations/Compare To Constant  relop=>=  const=0  OutDataTypeStr=boolean
  Demux : Demux
  w2 : Outport  VectorParamsAs1DForOutWhenUnconnected=off
  wires:
  w2_CMD/1 -> w2/1, Compare To Constant/1
  Compare To Constant/1 -> Demux/1
  Demux/1 -> Assertion/1
  Demux/4 -> Assertion3/1
  Demux/3 -> Assertion2/1
  Demux/2 -> Assertion1/1

== system bh_lag_LQI_eom_quad_include_spin_props/SAR/XYZ_CMDS ==
  Demux : Demux  Tag=STV Demux  Outputs=3
      settings: DisplayOption=none
  FromWs : FromWorkspace  Tag=STV FromWs  VariableName=tuvar
      SigBuilderData=|
      | common.afterFinalStr = 'Extrapolate'
      | common.sampleTime = 0
      | dataSet(1).timeRange = [0 200]
      | dataSet(1).name = 'small_steps'
      | dataSet(2).timeRange = [0 200]
      | dataSet(2).name = 'zStairs_xyConstVEL'
      | dataSet(3).timeRange = [0 500]
      | dataSet(3).name = 'sineWaves'
      | dataSet(4).timeRange = [0 200]
      | dataSet(4).name = 'ZERO'
      | dataSet(5).timeRange = [0 200]
      | dataSet(5).name = 'SEARCH_P1'
      | sbobj.Name = 'Signal Builder'
      | sbobj.Groups(1).Name = 'small_steps'
      | sbobj.Groups(1).Signals(1).Name = 'Z'
      | sbobj.Groups(1).Signals(1).XData = [0 10 10.000001 20 20.000001 30 30.000001 55 200]
      | sbobj.Groups(1).Signals(1).YData = [0 0 2 2 2 2 2 2 2]
      | sbobj.Groups(1).Signals(2).Name = 'X'
      | sbobj.Groups(1).Signals(2).XData = [0 10 10.000001 20 20.000001 30 30.000001 55 200]
      | sbobj.Groups(1).Signals(2).YData = [0 0 0 0 3 3 3 3 3]
      | sbobj.Groups(1).Signals(3).Name = 'Y'
      | sbobj.Groups(1).Signals(3).XData = [0 10 10.000001 20 20.000001 30 30.000001 55 200]
      | sbobj.Groups(1).Signals(3).YData = [0 0 0 0 0 0 1 1 1]
      | sbobj.Groups(1).TimeRange = [0 200]
      | sbobj.Groups(2).Name = 'zStairs_xyConstVEL'
      | sbobj.Groups(2).Signals(1).Name = 'Z'
      | sbobj.Groups(2).Signals(1).XData = [0 10 10.000001 20 20.000001 30 30.000001 40 40.000001 55 200]
      | sbobj.Groups(2).Signals(1).YData = [0 0 1 1 2 2 1 1 0 0 0]
      | sbobj.Groups(2).Signals(2).Name = 'X'
      | sbobj.Groups(2).Signals(2).XData = [0 10 10.000001 20 20.000001 30 30.000001 40 40.000001 55 200]
      | sbobj.Groups(2).Signals(2).YData = [0 1 1.0000001 2 2.0000001 3 3.0000001 4 4.0000001 5.5 20]
      | sbobj.Groups(2).Signals(3).Name = 'Y'
      | sbobj.Groups(2).Signals(3).XData = [0 10 10.000001 20 20.000001 30 30.000001 40 40.000001 55 200]
      | sbobj.Groups(2).Signals(3).YData = [0 0.5 0.50000005 1 1.00000005 1.5 1.50000005 2 2.00000005 2.75 10]
      | sbobj.Groups(2).TimeRange = [0 200]
      | sbobj.Groups(3).Name = 'sineWaves'
      | sbobj.Groups(3).Signals(1).Name = 'Z'
      | sbobj.Groups(3).Signals(1).XData = [0 0.1 0.2 0.3 0.4 0.5 0.6 0.7 0.8 0.9 1 1.1 ... (5001 elements, 1x5001)]
      | sbobj.Groups(3).Signals(1).YData = [0 0.0314107325553 0.0627904665622 0.0941082340641 0.125333128258 0.156434333994 0.18738115819 0.218143060119 0.248689681547 0.278990876699 0.309016742004 0.338737645607 ... (5001 elements, 1x5001)]
      | sbobj.Groups(3).Signals(2).Name = 'X'
      | sbobj.Groups(3).Signals(2).XData = [0 0.1 0.2 0.3 0.4 0.5 0.6 0.7 0.8 0.9 1 1.1 ... (5001 elements, 1x5001)]
      | sbobj.Groups(3).Signals(2).YData = [0 0.01 0.02 0.03 0.04 0.05 0.06 0.07 0.08 0.09 0.1 0.11 ... (5001 elements, 1x5001)]
      | sbobj.Groups(3).Signals(3).Name = 'Y'
      | sbobj.Groups(3).Signals(3).XData = [0 0.1 0.2 0.3 0.4 0.5 0.6 0.7 0.8 0.9 1 1.1 ... (5001 elements, 1x5001)]
      | sbobj.Groups(3).Signals(3).YData = [0 0.0157073040455 0.0314107325553 0.04710641095 0.0627904665622 0.0784590295926 0.0941082340641 0.109734218776 0.125333128258 0.140901113717 0.156434333994 0.171928956505 ... (5001 elements, 1x5001)]
      | sbobj.Groups(3).TimeRange = [0 500]
      | sbobj.Groups(4).Name = 'ZERO'
      | sbobj.Groups(4).Signals(1).Name = 'Z'
      | sbobj.Groups(4).Signals(1).XData = [0 200]
      | sbobj.Groups(4).Signals(1).YData = [0 0]
      | sbobj.Groups(4).Signals(2).Name = 'X'
      | sbobj.Groups(4).Signals(2).XData = [0 200]
      | sbobj.Groups(4).Signals(2).YData = [0 0]
      | sbobj.Groups(4).Signals(3).Name = 'Y'
      | sbobj.Groups(4).Signals(3).XData = [0 200]
      | sbobj.Groups(4).Signals(3).YData = [0 0]
      | sbobj.Groups(4).TimeRange = [0 200]
      | sbobj.Groups(5).Name = 'SEARCH_P1'
      | sbobj.Groups(5).Signals(1).Name = 'Z'
      | sbobj.Groups(5).Signals(1).XData = [0 7 27 32 52 57 77 82 102 107 127 132 157 187 200]
      | sbobj.Groups(5).Signals(1).YData = [0 5 5 5 5 5 5 5 5 5 5 5 5 0 0]
      | sbobj.Groups(5).Signals(2).Name = 'X'
      | sbobj.Groups(5).Signals(2).XData = [0 7 27 32 52 57 77 82 102 107 127 132 157 187 200]
      | sbobj.Groups(5).Signals(2).YData = [0 5 25 25 5 5 25 25 5 5 25 25 0 0 0]
      | sbobj.Groups(5).Signals(3).Name = 'Y'
      | sbobj.Groups(5).Signals(3).XData = [0 7 27 32 52 57 77 82 102 107 127 132 157 187 200]
      | sbobj.Groups(5).Signals(3).YData = [0 5 5 10 10 15 15 20 20 25 25 30 30 0 0]
      | sbobj.Groups(5).TimeRange = [0 200]
  Z : Outport  VectorParamsAs1DForOutWhenUnconnected=off
  X : Outport  Tag=STV Outport  Port=2  VectorParamsAs1DForOutWhenUnconnected=off
  Y : Outport  Tag=STV Outport  Port=3  VectorParamsAs1DForOutWhenUnconnected=off
  wires:
  Demux/1 -> Z/1
  FromWs/1 -> Demux/1
  Demux/2 -> X/1
  Demux/3 -> Y/1

== system bh_lag_LQI_eom_quad_include_spin_props/XYZ CMD_LIMITS/prefilter ==
  note: Y = U *     wn^2/( s^2 + 2*p*wn*s + wn^2)
      | Y*( s^2 + 2*p*wn*s + wn^2) = U * wn^2
      |
      | y'' + y'*2*p*wn + y*wn^2 = U*wn^2
  U : Inport
  Gain : Gain  Gain=2*p*wn
  Gain1 : Gain  Gain=wn^2
  Gain2 : Gain  Gain=wn^2
  Integrator : Integrator
  Integrator1 : Integrator
  Sum : Sum  Inputs=|+--
  U_filt : Outport  VectorParamsAs1DForOutWhenUnconnected=off
  U_DOT : Outport  Port=2  VectorParamsAs1DForOutWhenUnconnected=off
  wires:
  Integrator/1 -> Integrator1/1, [Y_DOT], Gain/1  "y_dot"
  Sum/1 -> Integrator/1  "y_dot_dot"
  Integrator1/1 -> Gain1/1, U_filt/1  "y"
  U/1 -> Gain2/1
  Gain2/1 -> Sum/1
  Gain/1 -> Sum/3
  Gain1/1 -> Sum/2
  [Y_DOT] -> U_DOT/1

== system bh_lag_LQI_eom_quad_include_spin_props/a_circle1/Signal Builder ==
  Demux : Demux  Tag=STV Demux  Outputs=2
      settings: DisplayOption=none
  FromWs : FromWorkspace  Tag=STV FromWs  VariableName=tuvar
      SigBuilderData=|
      | common.afterFinalStr = 'Extrapolate'
      | common.sampleTime = 0
      | dataSet.timeRange = [0 22]
      | dataSet.name = 'Group 1'
      | sbobj.Groups.Name = 'Group 1'
      | sbobj.Groups.Signals(1).Name = 'Signal 1'
      | sbobj.Groups.Signals(1).XData = [0 7.95 7.95 22]
      | sbobj.Groups.Signals(1).YData = [0 0 1.99 1.98]
      | sbobj.Groups.Signals(2).Name = 'Signal 2'
      | sbobj.Groups.Signals(2).XData = [0 12 16 22]
      | sbobj.Groups.Signals(2).YData = [0 0 1 1]
      | sbobj.Groups.TimeRange = [0 22]
  Signal 1 : Outport  Tag=STV Outport  VectorParamsAs1DForOutWhenUnconnected=off
  Signal 2 : Outport  Tag=STV Outport  Port=2  VectorParamsAs1DForOutWhenUnconnected=off
  wires:
  Demux/1 -> Signal 1/1
  FromWs/1 -> Demux/1
  Demux/2 -> Signal 2/1

== system bh_lag_LQI_eom_quad_include_spin_props/a_circle1/Subsystem ==
  RPS : Inport
  Constant : Constant  Value=2*pi
  Product : Product  Inputs=**
  w_rad_psec : Outport  VectorParamsAs1DForOutWhenUnconnected=off
  wires:
  Constant/1 -> Product/2
  RPS/1 -> Product/1
  Product/1 -> w_rad_psec/1

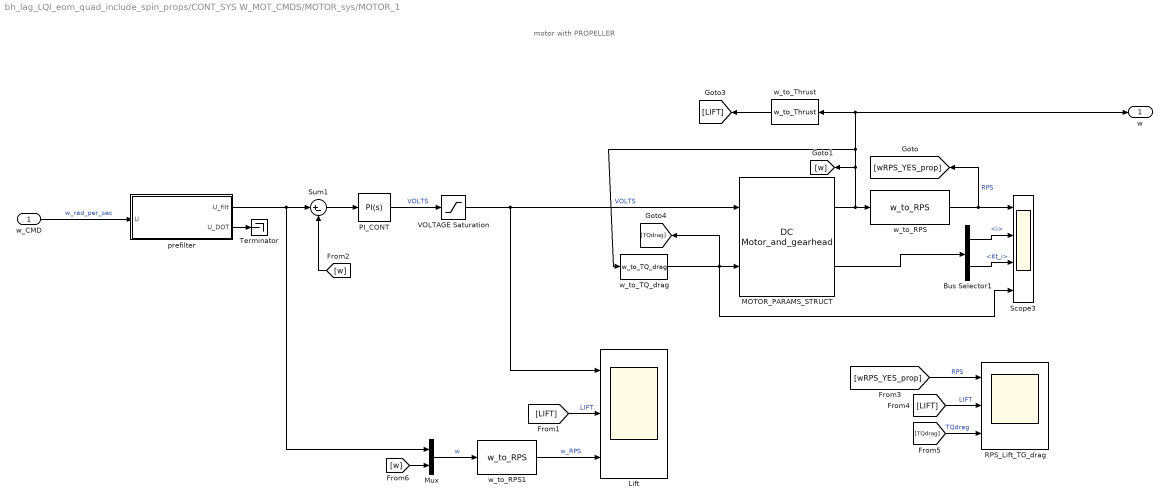
== system bh_lag_LQI_eom_quad_include_spin_props/CONT_SYS W_MOT_CMDS/MOTOR_sys/MOTOR_1 ==
  note: motor with PROPELLER
  w_CMD : Inport
  Bus Selector1 : BusSelector  OutputSignals=Elec.i,TQ_mot.Kt_i
  Lift : Scope  NumInputPorts=3
  MOTOR_PARAMS_STRUCT : bh_6dof_LIBRARY/MODELS/DC Motor_and_gearhead  K=P_mot.Ka  B=P_mot.b  J=P_mot.I  R=P_mot.R  L=P_mot.L  Kb=P_mot.Ke  ID=P_mot.ID
  Mux : Mux  Inputs=2
  PI_CONT : slpidlib/PID Controller  Controller=PI  Form=Parallel  TimeDomain=Continuous-time  UseExternalTs=off  SampleTime=-1  IntegratorMethod=Forward Euler  FilterMethod=Forward Euler  ControllerParametersSource=internal  P=2.97678216835849  I=24.9655384194189  D=-0.0417302954853434  UseFilter=on  N=6.67624174583517  TunerSelectOption=Transfer Function Based (PID Tuner App)  InitialConditionSource=internal  InitialConditionForIntegrator=0  InitialConditionForFilter=0  DifferentiatorICPrevScaledInput=0  ExternalReset=none  TrackingMode=off  Kt=1  LimitOutput=off  SatLimitsSource=internal  UpperSaturationLimit=inf  LowerSaturationLimit=-inf  LinearizeAsGain=on  AntiWindupMode=none  Kb=1  POutMin=[]  POutMax=[]  IOutMin=[]  IOutMax=[]  DOutMin=[]  DOutMax=[]  NOutMin=[]  NOutMax=[]  SumOutMin=[]  SumOutMax=[]  SaturationOutMin=[]  SaturationOutMax=[]  PParamMin=[]  PParamMax=[]  IParamMin=[]  IParamMax=[]  DParamMin=[]  DParamMax=[]  NParamMin=[]  NParamMax=[]  KbParamMin=[]  KbParamMax=[]  KtParamMin=[]  KtParamMax=[]  KbOutMin=[]  KbOutMax=[]  KtOutMin=[]  KtOutMax=[]  IntegratorOutMin=[]  IntegratorOutMax=[]  FilterOutMin=[]  FilterOutMax=[]  SumI1OutMin=[]  SumI1OutMax=[]  SumI2OutMin=[]  SumI2OutMax=[]  SumI3OutMin=[]  SumI3OutMax=[]  SumI4OutMin=[]  SumI4OutMax=[]  SumDOutMin=[]  SumDOutMax=[]  DifferentiatorOutMin=[]  DifferentiatorOutMax=[]  FilterDiffOutCoefMin=[]  FilterDiffOutCoefMax=[]  ReciprocalOutMin=[]  ReciprocalOutMax=[]  SumDenOutMin=[]  SumDenOutMax=[]  SumNumOutMin=[]  SumNumOutMax=[]  DivideOutMin=[]  DivideOutMax=[]  UdiffTsProdOutMin=[]  UdiffTsProdOutMax=[]  NTsProdOutMin=[]  NTsProdOutMax=[]  UintegralTsProdOutMin=[]  UintegralTsProdOutMax=[]  UngainTsProdOutMin=[]  UngainTsProdOutMax=[]  IntegratorContinuousStateAttributes=''  IntegratorStateMustResolveToSignalObject=off  IntegratorRTWStateStorageClass=Auto  FilterContinuousStateAttributes=''  FilterStateMustResolveToSignalObject=off  FilterRTWStateStorageClass=Auto  ParallelPVariant=InternalParameters  IdealPVariant=Disabled  IVariant=InternalParameters  DVariant=Disabled  IntegratorVariant=Continuous  SatVariant=Disabled  AWVariant=Passthrough  PCopyVariant=Disabled  TRVariant=Disabled  FdbkBlocksVariant=Forward  IdealPFdbkVariant=Disabled  SatFdbkVariant=Disabled  DerivativeFilterVariant=Disabled  NVariant=Disabled  NCopyVariant=Disabled_SignalSpec  FilterICVariant=Disabled  IntegratorICVariant=InternalICs  ExternalResetVariant=Disabled  TRSumVariant=Passthrough  SumFdbkVariant=Disabled  SumVariant=Sum_PI  TsampFilterVariant=InternalTs  TsampNgainVariant=Passthrough  TsampIntegralVariant=Passthrough  ExternalSaturationOutDataTypeStr=Inherit: Same as second input
  RPS_Lift_TG_drag : Scope  NumInputPorts=3
  Scope3 : Scope  NumInputPorts=4
  Sum1 : Sum  Inputs=|+-
  Terminator : Terminator
  VOLTAGE Saturation : Saturate  UpperLimit=P_elec.V_mot_max  LowerLimit=P_elec.V_mot_min
      settings: AttributesFormatString=|
      | Vmax = %<UpperLimit>
      | Vmin = %<LowerLimit>
  prefilter : Subsystem  mask(Derivative Estimation){wn=2*pi*5, p=1}
      mask prompts: wn "Natural frequency, wn (rad/sec)"; p "Damping ratio, p"
      mask help:
      | A simple derivative estimator using a 2nd order representation between input and output.
      |
      | The integrators use a discrete FORWARd Euler rule, and a sample time needs to be specified.
      mask init:
      | str1 = sprintf('wn = %.2f', wn);
      | str2 = sprintf('p  = %.2f', p);
      | %str3 = sprintf('dt = %.2f', dt);
      | %str = char(str1,str2,str3);
      | %str3 = sprintf('dt = %.2f', dt);
      | str = char(str1,str2);
      mask Display: disp(str)
  w_to_RPS : bh_6dof_LIBRARY/MODELS/w_to_RPS  SystemSampleTime=-1  VariantActivationTime=update diagram  Latency=0  AutoFrameSizeCalculation=off
  w_to_RPS1 : bh_6dof_LIBRARY/MODELS/w_to_RPS  SystemSampleTime=-1  VariantActivationTime=update diagram  Latency=0  AutoFrameSizeCalculation=off
  w_to_TQ_drag : bh_6dof_LIBRARY/MODELS/w_to_TQ_drag  k=P_one_prop.TWIST_per_w2
  w_to_Thrust : bh_6dof_LIBRARY/MODELS/w_to_Thrust  k=P_one_prop.LIFT_per_w2
  w : Outport  VectorParamsAs1DForOutWhenUnconnected=off
  wires:
  VOLTAGE Saturation/1 -> Lift/1, MOTOR_PARAMS_STRUCT/1  "VOLTS"
  [TQdrag] -> RPS_Lift_TG_drag/3  "TQdrag"
  Sum1/1 -> PI_CONT/1
  w_to_TQ_drag/1 -> [TQdrag], MOTOR_PARAMS_STRUCT/2, Scope3/4
  [LIFT] -> RPS_Lift_TG_drag/2  "LIFT"
  [wRPS_YES_prop] -> RPS_Lift_TG_drag/1  "RPS"
  w_to_Thrust/1 -> [LIFT]
  w_to_RPS/1 -> [wRPS_YES_prop], Scope3/1  "RPS"
  Bus Selector1/1 -> Scope3/2  "<i>"
  MOTOR_PARAMS_STRUCT/2 -> Bus Selector1/1
  Bus Selector1/2 -> Scope3/3  "<Kt_i>"
  MOTOR_PARAMS_STRUCT/1 -> w_to_RPS/1, [w], w/1, w_to_Thrust/1, w_to_TQ_drag/1
  [w] -> Sum1/2
  [LIFT] -> Lift/2  "LIFT"
  Mux/1 -> w_to_RPS1/1  "w"
  [w] -> Mux/2
  w_to_RPS1/1 -> Lift/3  "w_RPS"
  PI_CONT/1 -> VOLTAGE Saturation/1  "VOLTS"
  w_CMD/1 -> prefilter/1(U)  "w_rad_per_sec"
  prefilter/1(U_filt) -> Mux/1, Sum1/1
  prefilter/2(U_DOT) -> Terminator/1

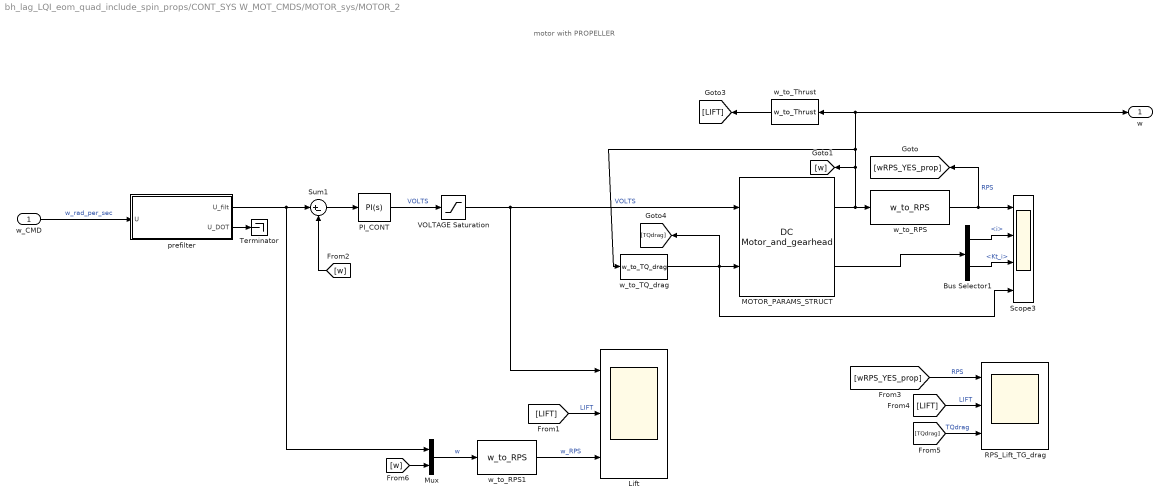
== system bh_lag_LQI_eom_quad_include_spin_props/CONT_SYS W_MOT_CMDS/MOTOR_sys/MOTOR_2 ==
  note: motor with PROPELLER
  w_CMD : Inport
  Bus Selector1 : BusSelector  OutputSignals=Elec.i,TQ_mot.Kt_i
  Lift : Scope  NumInputPorts=3
  MOTOR_PARAMS_STRUCT : bh_6dof_LIBRARY/MODELS/DC Motor_and_gearhead  K=P_mot.Ka  B=P_mot.b  J=P_mot.I  R=P_mot.R  L=P_mot.L  Kb=P_mot.Ke  ID=P_mot.ID
  Mux : Mux  Inputs=2
  PI_CONT : slpidlib/PID Controller  Controller=PI  Form=Parallel  TimeDomain=Continuous-time  UseExternalTs=off  SampleTime=-1  IntegratorMethod=Forward Euler  FilterMethod=Forward Euler  ControllerParametersSource=internal  P=2.97678216835849  I=24.9655384194189  D=-0.0417302954853434  UseFilter=on  N=6.67624174583517  TunerSelectOption=Transfer Function Based (PID Tuner App)  InitialConditionSource=internal  InitialConditionForIntegrator=0  InitialConditionForFilter=0  DifferentiatorICPrevScaledInput=0  ExternalReset=none  TrackingMode=off  Kt=1  LimitOutput=off  SatLimitsSource=internal  UpperSaturationLimit=inf  LowerSaturationLimit=-inf  LinearizeAsGain=on  AntiWindupMode=none  Kb=1  POutMin=[]  POutMax=[]  IOutMin=[]  IOutMax=[]  DOutMin=[]  DOutMax=[]  NOutMin=[]  NOutMax=[]  SumOutMin=[]  SumOutMax=[]  SaturationOutMin=[]  SaturationOutMax=[]  PParamMin=[]  PParamMax=[]  IParamMin=[]  IParamMax=[]  DParamMin=[]  DParamMax=[]  NParamMin=[]  NParamMax=[]  KbParamMin=[]  KbParamMax=[]  KtParamMin=[]  KtParamMax=[]  KbOutMin=[]  KbOutMax=[]  KtOutMin=[]  KtOutMax=[]  IntegratorOutMin=[]  IntegratorOutMax=[]  FilterOutMin=[]  FilterOutMax=[]  SumI1OutMin=[]  SumI1OutMax=[]  SumI2OutMin=[]  SumI2OutMax=[]  SumI3OutMin=[]  SumI3OutMax=[]  SumI4OutMin=[]  SumI4OutMax=[]  SumDOutMin=[]  SumDOutMax=[]  DifferentiatorOutMin=[]  DifferentiatorOutMax=[]  FilterDiffOutCoefMin=[]  FilterDiffOutCoefMax=[]  ReciprocalOutMin=[]  ReciprocalOutMax=[]  SumDenOutMin=[]  SumDenOutMax=[]  SumNumOutMin=[]  SumNumOutMax=[]  DivideOutMin=[]  DivideOutMax=[]  UdiffTsProdOutMin=[]  UdiffTsProdOutMax=[]  NTsProdOutMin=[]  NTsProdOutMax=[]  UintegralTsProdOutMin=[]  UintegralTsProdOutMax=[]  UngainTsProdOutMin=[]  UngainTsProdOutMax=[]  IntegratorContinuousStateAttributes=''  IntegratorStateMustResolveToSignalObject=off  IntegratorRTWStateStorageClass=Auto  FilterContinuousStateAttributes=''  FilterStateMustResolveToSignalObject=off  FilterRTWStateStorageClass=Auto  ParallelPVariant=InternalParameters  IdealPVariant=Disabled  IVariant=InternalParameters  DVariant=Disabled  IntegratorVariant=Continuous  SatVariant=Disabled  AWVariant=Passthrough  PCopyVariant=Disabled  TRVariant=Disabled  FdbkBlocksVariant=Forward  IdealPFdbkVariant=Disabled  SatFdbkVariant=Disabled  DerivativeFilterVariant=Disabled  NVariant=Disabled  NCopyVariant=Disabled_SignalSpec  FilterICVariant=Disabled  IntegratorICVariant=InternalICs  ExternalResetVariant=Disabled  TRSumVariant=Passthrough  SumFdbkVariant=Disabled  SumVariant=Sum_PI  TsampFilterVariant=InternalTs  TsampNgainVariant=Passthrough  TsampIntegralVariant=Passthrough  ExternalSaturationOutDataTypeStr=Inherit: Same as second input
  RPS_Lift_TG_drag : Scope  NumInputPorts=3
  Scope3 : Scope  NumInputPorts=4
  Sum1 : Sum  Inputs=|+-
  Terminator : Terminator
  VOLTAGE Saturation : Saturate  UpperLimit=P_elec.V_mot_max  LowerLimit=P_elec.V_mot_min
      settings: AttributesFormatString=|
      | Vmax = %<UpperLimit>
      | Vmin = %<LowerLimit>
  prefilter : Subsystem  mask(Derivative Estimation){wn=2*pi*5, p=1}
      mask prompts: wn "Natural frequency, wn (rad/sec)"; p "Damping ratio, p"
      mask help:
      | A simple derivative estimator using a 2nd order representation between input and output.
      |
      | The integrators use a discrete FORWARd Euler rule, and a sample time needs to be specified.
      mask init:
      | str1 = sprintf('wn = %.2f', wn);
      | str2 = sprintf('p  = %.2f', p);
      | %str3 = sprintf('dt = %.2f', dt);
      | %str = char(str1,str2,str3);
      | %str3 = sprintf('dt = %.2f', dt);
      | str = char(str1,str2);
      mask Display: disp(str)
  w_to_RPS : bh_6dof_LIBRARY/MODELS/w_to_RPS  SystemSampleTime=-1  VariantActivationTime=update diagram  Latency=0  AutoFrameSizeCalculation=off
  w_to_RPS1 : bh_6dof_LIBRARY/MODELS/w_to_RPS  SystemSampleTime=-1  VariantActivationTime=update diagram  Latency=0  AutoFrameSizeCalculation=off
  w_to_TQ_drag : bh_6dof_LIBRARY/MODELS/w_to_TQ_drag  k=P_one_prop.TWIST_per_w2
  w_to_Thrust : bh_6dof_LIBRARY/MODELS/w_to_Thrust  k=P_one_prop.LIFT_per_w2
  w : Outport  VectorParamsAs1DForOutWhenUnconnected=off
  wires:
  VOLTAGE Saturation/1 -> Lift/1, MOTOR_PARAMS_STRUCT/1  "VOLTS"
  [TQdrag] -> RPS_Lift_TG_drag/3  "TQdrag"
  Sum1/1 -> PI_CONT/1
  w_to_TQ_drag/1 -> [TQdrag], MOTOR_PARAMS_STRUCT/2, Scope3/4
  [LIFT] -> RPS_Lift_TG_drag/2  "LIFT"
  [wRPS_YES_prop] -> RPS_Lift_TG_drag/1  "RPS"
  w_to_Thrust/1 -> [LIFT]
  w_to_RPS/1 -> [wRPS_YES_prop], Scope3/1  "RPS"
  Bus Selector1/1 -> Scope3/2  "<i>"
  MOTOR_PARAMS_STRUCT/2 -> Bus Selector1/1
  Bus Selector1/2 -> Scope3/3  "<Kt_i>"
  MOTOR_PARAMS_STRUCT/1 -> w_to_RPS/1, [w], w/1, w_to_Thrust/1, w_to_TQ_drag/1
  [w] -> Sum1/2
  [LIFT] -> Lift/2  "LIFT"
  Mux/1 -> w_to_RPS1/1  "w"
  [w] -> Mux/2
  w_to_RPS1/1 -> Lift/3  "w_RPS"
  PI_CONT/1 -> VOLTAGE Saturation/1  "VOLTS"
  w_CMD/1 -> prefilter/1(U)  "w_rad_per_sec"
  prefilter/1(U_filt) -> Mux/1, Sum1/1
  prefilter/2(U_DOT) -> Terminator/1

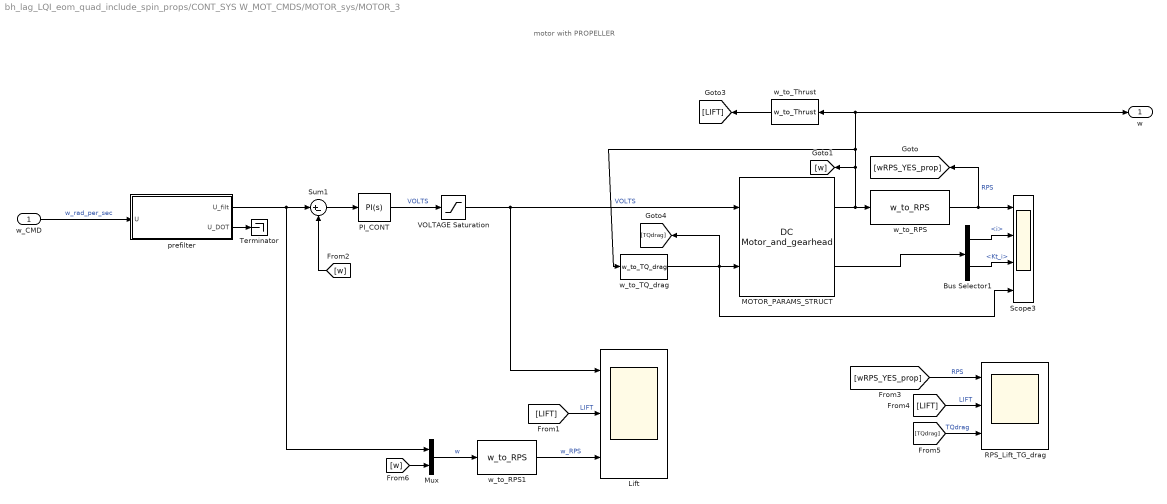
== system bh_lag_LQI_eom_quad_include_spin_props/CONT_SYS W_MOT_CMDS/MOTOR_sys/MOTOR_3 ==
  note: motor with PROPELLER
  w_CMD : Inport
  Bus Selector1 : BusSelector  OutputSignals=Elec.i,TQ_mot.Kt_i
  Lift : Scope  NumInputPorts=3
  MOTOR_PARAMS_STRUCT : bh_6dof_LIBRARY/MODELS/DC Motor_and_gearhead  K=P_mot.Ka  B=P_mot.b  J=P_mot.I  R=P_mot.R  L=P_mot.L  Kb=P_mot.Ke  ID=P_mot.ID
  Mux : Mux  Inputs=2
  PI_CONT : slpidlib/PID Controller  Controller=PI  Form=Parallel  TimeDomain=Continuous-time  UseExternalTs=off  SampleTime=-1  IntegratorMethod=Forward Euler  FilterMethod=Forward Euler  ControllerParametersSource=internal  P=2.97678216835849  I=24.9655384194189  D=-0.0417302954853434  UseFilter=on  N=6.67624174583517  TunerSelectOption=Transfer Function Based (PID Tuner App)  InitialConditionSource=internal  InitialConditionForIntegrator=0  InitialConditionForFilter=0  DifferentiatorICPrevScaledInput=0  ExternalReset=none  TrackingMode=off  Kt=1  LimitOutput=off  SatLimitsSource=internal  UpperSaturationLimit=inf  LowerSaturationLimit=-inf  LinearizeAsGain=on  AntiWindupMode=none  Kb=1  POutMin=[]  POutMax=[]  IOutMin=[]  IOutMax=[]  DOutMin=[]  DOutMax=[]  NOutMin=[]  NOutMax=[]  SumOutMin=[]  SumOutMax=[]  SaturationOutMin=[]  SaturationOutMax=[]  PParamMin=[]  PParamMax=[]  IParamMin=[]  IParamMax=[]  DParamMin=[]  DParamMax=[]  NParamMin=[]  NParamMax=[]  KbParamMin=[]  KbParamMax=[]  KtParamMin=[]  KtParamMax=[]  KbOutMin=[]  KbOutMax=[]  KtOutMin=[]  KtOutMax=[]  IntegratorOutMin=[]  IntegratorOutMax=[]  FilterOutMin=[]  FilterOutMax=[]  SumI1OutMin=[]  SumI1OutMax=[]  SumI2OutMin=[]  SumI2OutMax=[]  SumI3OutMin=[]  SumI3OutMax=[]  SumI4OutMin=[]  SumI4OutMax=[]  SumDOutMin=[]  SumDOutMax=[]  DifferentiatorOutMin=[]  DifferentiatorOutMax=[]  FilterDiffOutCoefMin=[]  FilterDiffOutCoefMax=[]  ReciprocalOutMin=[]  ReciprocalOutMax=[]  SumDenOutMin=[]  SumDenOutMax=[]  SumNumOutMin=[]  SumNumOutMax=[]  DivideOutMin=[]  DivideOutMax=[]  UdiffTsProdOutMin=[]  UdiffTsProdOutMax=[]  NTsProdOutMin=[]  NTsProdOutMax=[]  UintegralTsProdOutMin=[]  UintegralTsProdOutMax=[]  UngainTsProdOutMin=[]  UngainTsProdOutMax=[]  IntegratorContinuousStateAttributes=''  IntegratorStateMustResolveToSignalObject=off  IntegratorRTWStateStorageClass=Auto  FilterContinuousStateAttributes=''  FilterStateMustResolveToSignalObject=off  FilterRTWStateStorageClass=Auto  ParallelPVariant=InternalParameters  IdealPVariant=Disabled  IVariant=InternalParameters  DVariant=Disabled  IntegratorVariant=Continuous  SatVariant=Disabled  AWVariant=Passthrough  PCopyVariant=Disabled  TRVariant=Disabled  FdbkBlocksVariant=Forward  IdealPFdbkVariant=Disabled  SatFdbkVariant=Disabled  DerivativeFilterVariant=Disabled  NVariant=Disabled  NCopyVariant=Disabled_SignalSpec  FilterICVariant=Disabled  IntegratorICVariant=InternalICs  ExternalResetVariant=Disabled  TRSumVariant=Passthrough  SumFdbkVariant=Disabled  SumVariant=Sum_PI  TsampFilterVariant=InternalTs  TsampNgainVariant=Passthrough  TsampIntegralVariant=Passthrough  ExternalSaturationOutDataTypeStr=Inherit: Same as second input
  RPS_Lift_TG_drag : Scope  NumInputPorts=3
  Scope3 : Scope  NumInputPorts=4
  Sum1 : Sum  Inputs=|+-
  Terminator : Terminator
  VOLTAGE Saturation : Saturate  UpperLimit=P_elec.V_mot_max  LowerLimit=P_elec.V_mot_min
      settings: AttributesFormatString=|
      | Vmax = %<UpperLimit>
      | Vmin = %<LowerLimit>
  prefilter : Subsystem  mask(Derivative Estimation){wn=2*pi*5, p=1}
      mask prompts: wn "Natural frequency, wn (rad/sec)"; p "Damping ratio, p"
      mask help:
      | A simple derivative estimator using a 2nd order representation between input and output.
      |
      | The integrators use a discrete FORWARd Euler rule, and a sample time needs to be specified.
      mask init:
      | str1 = sprintf('wn = %.2f', wn);
      | str2 = sprintf('p  = %.2f', p);
      | %str3 = sprintf('dt = %.2f', dt);
      | %str = char(str1,str2,str3);
      | %str3 = sprintf('dt = %.2f', dt);
      | str = char(str1,str2);
      mask Display: disp(str)
  w_to_RPS : bh_6dof_LIBRARY/MODELS/w_to_RPS  SystemSampleTime=-1  VariantActivationTime=update diagram  Latency=0  AutoFrameSizeCalculation=off
  w_to_RPS1 : bh_6dof_LIBRARY/MODELS/w_to_RPS  SystemSampleTime=-1  VariantActivationTime=update diagram  Latency=0  AutoFrameSizeCalculation=off
  w_to_TQ_drag : bh_6dof_LIBRARY/MODELS/w_to_TQ_drag  k=P_one_prop.TWIST_per_w2
  w_to_Thrust : bh_6dof_LIBRARY/MODELS/w_to_Thrust  k=P_one_prop.LIFT_per_w2
  w : Outport  VectorParamsAs1DForOutWhenUnconnected=off
  wires:
  VOLTAGE Saturation/1 -> Lift/1, MOTOR_PARAMS_STRUCT/1  "VOLTS"
  [TQdrag] -> RPS_Lift_TG_drag/3  "TQdrag"
  Sum1/1 -> PI_CONT/1
  w_to_TQ_drag/1 -> [TQdrag], MOTOR_PARAMS_STRUCT/2, Scope3/4
  [LIFT] -> RPS_Lift_TG_drag/2  "LIFT"
  [wRPS_YES_prop] -> RPS_Lift_TG_drag/1  "RPS"
  w_to_Thrust/1 -> [LIFT]
  w_to_RPS/1 -> [wRPS_YES_prop], Scope3/1  "RPS"
  Bus Selector1/1 -> Scope3/2  "<i>"
  MOTOR_PARAMS_STRUCT/2 -> Bus Selector1/1
  Bus Selector1/2 -> Scope3/3  "<Kt_i>"
  MOTOR_PARAMS_STRUCT/1 -> w_to_RPS/1, [w], w/1, w_to_Thrust/1, w_to_TQ_drag/1
  [w] -> Sum1/2
  [LIFT] -> Lift/2  "LIFT"
  Mux/1 -> w_to_RPS1/1  "w"
  [w] -> Mux/2
  w_to_RPS1/1 -> Lift/3  "w_RPS"
  PI_CONT/1 -> VOLTAGE Saturation/1  "VOLTS"
  w_CMD/1 -> prefilter/1(U)  "w_rad_per_sec"
  prefilter/1(U_filt) -> Mux/1, Sum1/1
  prefilter/2(U_DOT) -> Terminator/1

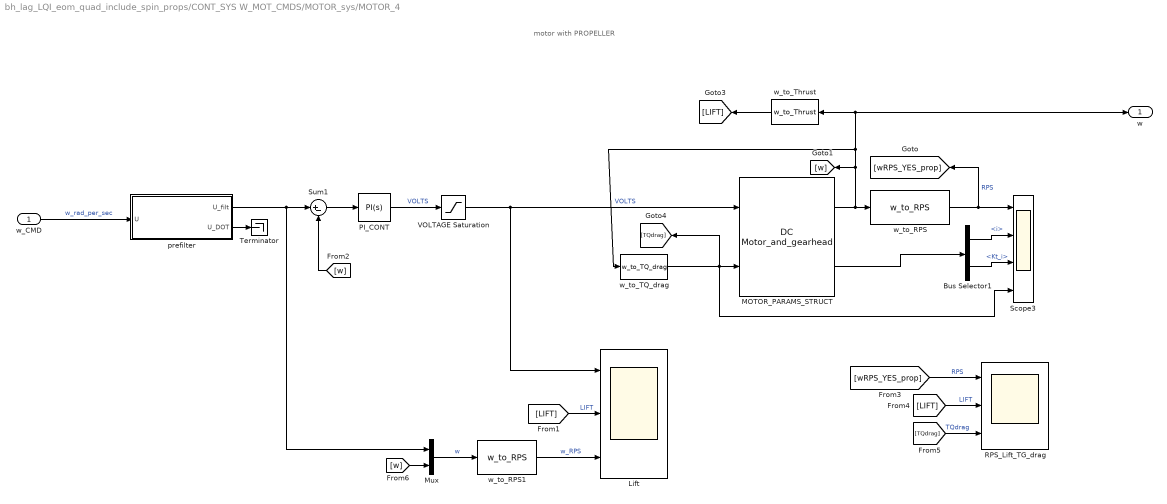
== system bh_lag_LQI_eom_quad_include_spin_props/CONT_SYS W_MOT_CMDS/MOTOR_sys/MOTOR_4 ==
  note: motor with PROPELLER
  w_CMD : Inport
  Bus Selector1 : BusSelector  OutputSignals=Elec.i,TQ_mot.Kt_i
  Lift : Scope  NumInputPorts=3
  MOTOR_PARAMS_STRUCT : bh_6dof_LIBRARY/MODELS/DC Motor_and_gearhead  K=P_mot.Ka  B=P_mot.b  J=P_mot.I  R=P_mot.R  L=P_mot.L  Kb=P_mot.Ke  ID=P_mot.ID
  Mux : Mux  Inputs=2
  PI_CONT : slpidlib/PID Controller  Controller=PI  Form=Parallel  TimeDomain=Continuous-time  UseExternalTs=off  SampleTime=-1  IntegratorMethod=Forward Euler  FilterMethod=Forward Euler  ControllerParametersSource=internal  P=2.97678216835849  I=24.9655384194189  D=-0.0417302954853434  UseFilter=on  N=6.67624174583517  TunerSelectOption=Transfer Function Based (PID Tuner App)  InitialConditionSource=internal  InitialConditionForIntegrator=0  InitialConditionForFilter=0  DifferentiatorICPrevScaledInput=0  ExternalReset=none  TrackingMode=off  Kt=1  LimitOutput=off  SatLimitsSource=internal  UpperSaturationLimit=inf  LowerSaturationLimit=-inf  LinearizeAsGain=on  AntiWindupMode=none  Kb=1  POutMin=[]  POutMax=[]  IOutMin=[]  IOutMax=[]  DOutMin=[]  DOutMax=[]  NOutMin=[]  NOutMax=[]  SumOutMin=[]  SumOutMax=[]  SaturationOutMin=[]  SaturationOutMax=[]  PParamMin=[]  PParamMax=[]  IParamMin=[]  IParamMax=[]  DParamMin=[]  DParamMax=[]  NParamMin=[]  NParamMax=[]  KbParamMin=[]  KbParamMax=[]  KtParamMin=[]  KtParamMax=[]  KbOutMin=[]  KbOutMax=[]  KtOutMin=[]  KtOutMax=[]  IntegratorOutMin=[]  IntegratorOutMax=[]  FilterOutMin=[]  FilterOutMax=[]  SumI1OutMin=[]  SumI1OutMax=[]  SumI2OutMin=[]  SumI2OutMax=[]  SumI3OutMin=[]  SumI3OutMax=[]  SumI4OutMin=[]  SumI4OutMax=[]  SumDOutMin=[]  SumDOutMax=[]  DifferentiatorOutMin=[]  DifferentiatorOutMax=[]  FilterDiffOutCoefMin=[]  FilterDiffOutCoefMax=[]  ReciprocalOutMin=[]  ReciprocalOutMax=[]  SumDenOutMin=[]  SumDenOutMax=[]  SumNumOutMin=[]  SumNumOutMax=[]  DivideOutMin=[]  DivideOutMax=[]  UdiffTsProdOutMin=[]  UdiffTsProdOutMax=[]  NTsProdOutMin=[]  NTsProdOutMax=[]  UintegralTsProdOutMin=[]  UintegralTsProdOutMax=[]  UngainTsProdOutMin=[]  UngainTsProdOutMax=[]  IntegratorContinuousStateAttributes=''  IntegratorStateMustResolveToSignalObject=off  IntegratorRTWStateStorageClass=Auto  FilterContinuousStateAttributes=''  FilterStateMustResolveToSignalObject=off  FilterRTWStateStorageClass=Auto  ParallelPVariant=InternalParameters  IdealPVariant=Disabled  IVariant=InternalParameters  DVariant=Disabled  IntegratorVariant=Continuous  SatVariant=Disabled  AWVariant=Passthrough  PCopyVariant=Disabled  TRVariant=Disabled  FdbkBlocksVariant=Forward  IdealPFdbkVariant=Disabled  SatFdbkVariant=Disabled  DerivativeFilterVariant=Disabled  NVariant=Disabled  NCopyVariant=Disabled_SignalSpec  FilterICVariant=Disabled  IntegratorICVariant=InternalICs  ExternalResetVariant=Disabled  TRSumVariant=Passthrough  SumFdbkVariant=Disabled  SumVariant=Sum_PI  TsampFilterVariant=InternalTs  TsampNgainVariant=Passthrough  TsampIntegralVariant=Passthrough  ExternalSaturationOutDataTypeStr=Inherit: Same as second input
  RPS_Lift_TG_drag : Scope  NumInputPorts=3
  Scope3 : Scope  NumInputPorts=4
  Sum1 : Sum  Inputs=|+-
  Terminator : Terminator
  VOLTAGE Saturation : Saturate  UpperLimit=P_elec.V_mot_max  LowerLimit=P_elec.V_mot_min
      settings: AttributesFormatString=|
      | Vmax = %<UpperLimit>
      | Vmin = %<LowerLimit>
  prefilter : Subsystem  mask(Derivative Estimation){wn=2*pi*5, p=1}
      mask prompts: wn "Natural frequency, wn (rad/sec)"; p "Damping ratio, p"
      mask help:
      | A simple derivative estimator using a 2nd order representation between input and output.
      |
      | The integrators use a discrete FORWARd Euler rule, and a sample time needs to be specified.
      mask init:
      | str1 = sprintf('wn = %.2f', wn);
      | str2 = sprintf('p  = %.2f', p);
      | %str3 = sprintf('dt = %.2f', dt);
      | %str = char(str1,str2,str3);
      | %str3 = sprintf('dt = %.2f', dt);
      | str = char(str1,str2);
      mask Display: disp(str)
  w_to_RPS : bh_6dof_LIBRARY/MODELS/w_to_RPS  SystemSampleTime=-1  VariantActivationTime=update diagram  Latency=0  AutoFrameSizeCalculation=off
  w_to_RPS1 : bh_6dof_LIBRARY/MODELS/w_to_RPS  SystemSampleTime=-1  VariantActivationTime=update diagram  Latency=0  AutoFrameSizeCalculation=off
  w_to_TQ_drag : bh_6dof_LIBRARY/MODELS/w_to_TQ_drag  k=P_one_prop.TWIST_per_w2
  w_to_Thrust : bh_6dof_LIBRARY/MODELS/w_to_Thrust  k=P_one_prop.LIFT_per_w2
  w : Outport  VectorParamsAs1DForOutWhenUnconnected=off
  wires:
  VOLTAGE Saturation/1 -> Lift/1, MOTOR_PARAMS_STRUCT/1  "VOLTS"
  [TQdrag] -> RPS_Lift_TG_drag/3  "TQdrag"
  Sum1/1 -> PI_CONT/1
  w_to_TQ_drag/1 -> [TQdrag], MOTOR_PARAMS_STRUCT/2, Scope3/4
  [LIFT] -> RPS_Lift_TG_drag/2  "LIFT"
  [wRPS_YES_prop] -> RPS_Lift_TG_drag/1  "RPS"
  w_to_Thrust/1 -> [LIFT]
  w_to_RPS/1 -> [wRPS_YES_prop], Scope3/1  "RPS"
  Bus Selector1/1 -> Scope3/2  "<i>"
  MOTOR_PARAMS_STRUCT/2 -> Bus Selector1/1
  Bus Selector1/2 -> Scope3/3  "<Kt_i>"
  MOTOR_PARAMS_STRUCT/1 -> w_to_RPS/1, [w], w/1, w_to_Thrust/1, w_to_TQ_drag/1
  [w] -> Sum1/2
  [LIFT] -> Lift/2  "LIFT"
  Mux/1 -> w_to_RPS1/1  "w"
  [w] -> Mux/2
  w_to_RPS1/1 -> Lift/3  "w_RPS"
  PI_CONT/1 -> VOLTAGE Saturation/1  "VOLTS"
  w_CMD/1 -> prefilter/1(U)  "w_rad_per_sec"
  prefilter/1(U_filt) -> Mux/1, Sum1/1
  prefilter/2(U_DOT) -> Terminator/1
